simulink model "es_tipo_esame_2_schema"  (R2021b)
settings: Solver=VariableStepAuto  StartTime=0.0  StopTime=50  RelTol=1e-3
values from neighbouring files (symbols this model uses):
  Kr = 1    [L_11_05_21_reti_anticipatrici.m]    (also in L_11_05_21_reti_anticipatrici_2.m; L_12_05_21_Esercizio_progetto_di_un_controllore.m; L_12_05_21_effetti_sul_comando.m; L_12_05_21_reti_integro-derivative.m)
  s = tf('s')    [L_04_05_21_es_stabilita_marginale.m]    (also in L_11_05_21_reti_anticipatrici.m; L_11_05_21_reti_anticipatrici_2.m; L_12_05_21_Esercizio_progetto_di_un_controllore.m; L_12_05_21_effetti_sul_comando.m)
libraries: cstblocks x4, simulink x1
settings Model: Creator=francescafornasier  LastModifiedBy=francescafornasier

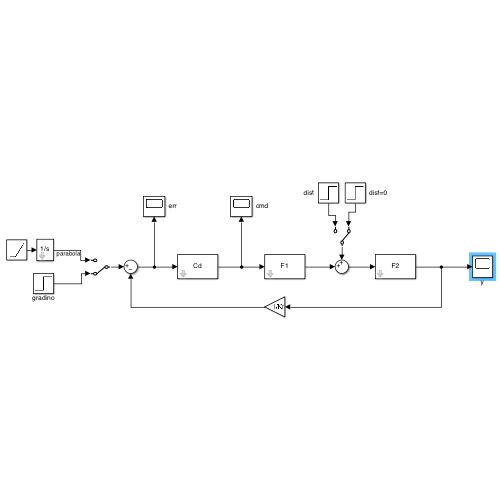
[thumbnail: Simulink's stored preview of the top-level diagram]
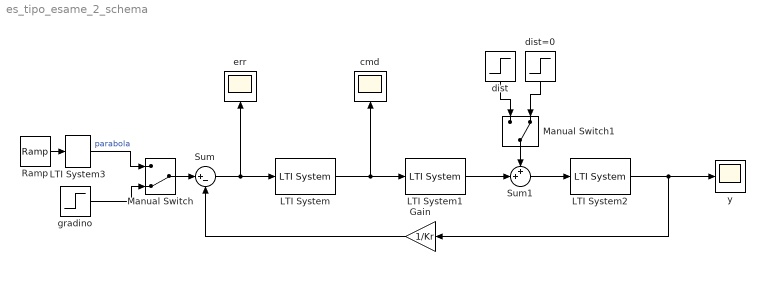
== system es_tipo_esame_2_schema ==
  Gain : Gain  Gain=1/Kr
  LTI System : cstblocks/LTI System  sys=Cd  IC=[]
  LTI System1 : cstblocks/LTI System  sys=F1  IC=[]
  LTI System2 : cstblocks/LTI System  sys=F2  IC=[]
  LTI System3 : cstblocks/LTI System  sys=1/s  IC=[]
  Manual Switch : ManualSwitch  CurrentSetting=0
  Manual Switch1 : ManualSwitch  CurrentSetting=0
  Ramp : simulink/Sources/Ramp  slope=1  start=0  InitialOutput=0
  Sum : Sum  Inputs=|+-
  Sum1 : Sum  Inputs=++|
  cmd : Scope
  dist : Step  Time=0  After=1.5  SampleTime=0
  dist=0 : Step  Time=0  After=0  SampleTime=0
  err : Scope
  gradino : Step  Time=0  SampleTime=0
  y : Scope
  wires:
  Manual Switch/1 -> Sum/1
  LTI System3/1 -> Manual Switch/1  "parabola"
  gradino/1 -> Manual Switch/2
  Gain/1 -> Sum/2
  Sum/1 -> LTI System/1, err/1
  LTI System1/1 -> Sum1/2
  Sum1/1 -> LTI System2/1
  LTI System2/1 -> y/1, Gain/1
  LTI System/1 -> cmd/1, LTI System1/1
  Manual Switch1/1 -> Sum1/1
  dist/1 -> Manual Switch1/1
  dist=0/1 -> Manual Switch1/2
  Ramp/1 -> LTI System3/1
